simulink model "Model"  (R2023b)
settings: Solver=ode4  StartTime=0.0  StopTime=inf  FixedStep=1e-3  RelTol=1e-3
undefined symbols (not defined in the file): Actuatorparams, Aeroparams, Aircraftparams, Atmosphereparams, Earth, Inertiaconstants, Initialconds, Propparams, WGS84
libraries: simulink_extras x29, aerolibfltsims x2, aerolibtransform2 x1, vrlib x1
(part 1 of 3)
settings Model: Creator=bilal  LastModifiedBy=bilal
settings DebuggingCC: BusObjectLabelMismatch=error

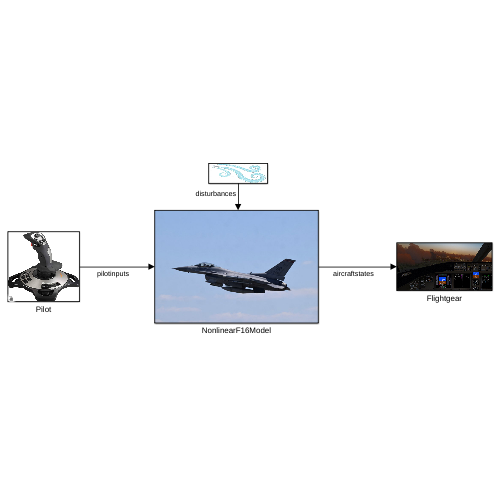
[thumbnail: Simulink's stored preview of the top-level diagram]
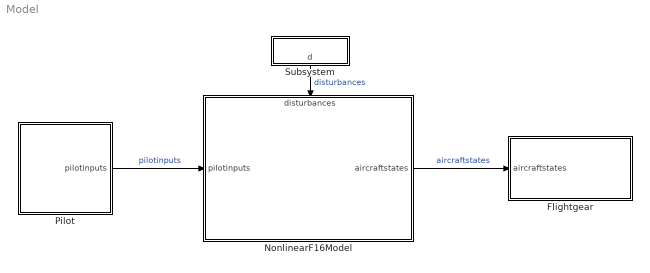
== system Model ==
  Flightgear : Subsystem
      mask Display: image('flightgear.jpg');
  NonlinearF16Model : Subsystem
      settings: PortSchema="{\"entries\":[{\"content\":{\"sides\":[{\"content\":{\"connectorIds\":[\"In1\"]},\"type\":\"ConnectorPlacement.EquallySpacedRectSide\",\"uuid\":\"b6fae004-6bc9-43de-a584-fcbf29e22be7\"},{\"content\":{\"connectorIds\":[\"Out1\"],\"side\":\"RIGHT\"},\"type\":\"ConnectorPlacement.EquallySpacedRectSide\",\"uuid\":\"50eeeff7-cc9e-45ad-978f-3a1c4ba7fd3d\"},{\"content\":{\"connectorIds\":[\"In2\"],\"side\":\"TOP\"},\"type\":\"ConnectorPlacement.EquallySpacedRectSide\",\"uuid\":\"669eaa38-3e90-4fd8-9c1d-c16541f97941\"}]},\"type\":\"ConnectorPlacement.EquallySpacedConnector\",\"uuid\":\"be7d5b6d-756e-471d-af56-7628ad948b10\"}],\"packageUris\":[\"http://schema.mathworks.com/mf0/Connector/R2020b\"],\"version\":\"1.0\"}"
      mask Display: image('f16.jpg');
  Pilot : Subsystem  Variant=on  VariantControlMode=label  LabelModeActiveChoice=pilotmode=manual
      mask Display: image('joystick.jpg');
  Subsystem : Subsystem
      mask Display: image('disturbance.png');
  wires:
  Pilot/1(pilotinputs) -> NonlinearF16Model/1(pilotinputs)  "pilotinputs"
  Subsystem/1(d) -> NonlinearF16Model/2(disturbances)  "disturbances"
  NonlinearF16Model/1(aircraftstates) -> Flightgear/1(aircraftstates)  "aircraftstates"

== system Model/Flightgear ==
  note: Instructions to setup FlightGear
      | Install FlightGear .
      | Open 'Generate Run Script' on the right.
      | On the Flightgear tab type your aircraft model name in 'FlightGear geometry model name'.
      | - Recommended model: 'c172p' as FlightGear
      | installes it by default.
      | - Additional aircrafts can be downloaded then.
      | On the File FlightGear base directory.
      | Click Generate Script.
      | Run generated script in Command Prompt (Windows) or in Terminal (Linux/macOS).
  aircraftstates : Inport
  Bus Selector : BusSelector  OutputSignals=rigidbodystates.positions.xe,rigidbodystates.positions.ye,rigidbodystates.positions.ze,rigidbodystates.eulerangles.phi,rigidbodystates.eulerangles.theta,rigidbodystates.eulerangles.psi
  Constant : Constant  Value=Initialconds.zeic
  Demux : Demux  Outputs=2
  Flat Earth to LLA : aerolibtransform2/Flat Earth to LLA  units=Metric (MKS)  ptype=Earth (WGS84)  F=1/298.257223563  R=6378137  refPosPort=off  LL0=[0 10]  psi=0
  FlightGear Preconfigured 6DoF Animation : aerolibfltsims/FlightGear Preconfigured 6DoF Animation  xFlightGearVersion=v2019.1  DestinationIpAddress=127.0.0.1  DestinationPort=5502  SampleTime=1e-3  packetVersion=24
  Flip : DSPFlip
  Generate Run Script : aerolibfltsims/Generate Run Script  Architecture=Default  dataFlow=Send  GeometryModelName=c172p  AirportId=KSFO  RunwayId=10L  InitialAltitude=7224  InitialHeading=113  OffsetDistance=4.72  OffsetAzimuth=0  InstallScenery=off  DisableShaders=off  OriginAddress=127.0.0.1  DestinationPort=5502  OriginPort=5505  LocalAddress=127.0.0.1  OutputFileName=runfg.bat  FlightGearBaseDirectory=C:\Program Files\FlightGear
  Mux : Mux  Inputs=3
  Mux1 : Mux  Inputs=6
  wires:
  aircraftstates/1 -> Bus Selector/1
  Bus Selector/2 -> Mux/2  "<ye>"
  Bus Selector/1 -> Mux/1  "<xe>"
  Bus Selector/3 -> Mux/3  "<ze>"
  Mux/1 -> Flat Earth to LLA/1
  Bus Selector/4 -> Mux1/4  "<phi>"
  Bus Selector/5 -> Mux1/5  "<theta>"
  Bus Selector/6 -> Mux1/6  "<psi>"
  Flat Earth to LLA/1 -> Flip/1
  Flip/1 -> Demux/1
  Demux/1 -> Mux1/1
  Demux/2 -> Mux1/2
  Flat Earth to LLA/2 -> Mux1/3
  Mux1/1 -> FlightGear Preconfigured 6DoF Animation/1
  Constant/1 -> Flat Earth to LLA/2

== system Model/NonlinearF16Model ==
  pilotinputs : Inport  OutDataTypeStr=Bus: pilotinputs
  disturbances : Inport  Port=2  OutDataTypeStr=Bus: disturbances
  Airframe : Subsystem
  Simframe : Subsystem
  aircraftstates : Outport  OutDataTypeStr=Bus: aircraftstates
  wires:
  pilotinputs/1 -> Airframe/1(pilotinputs)  "pilotinputs"
  Airframe/1(totalforces) -> Simframe/1(totalforces)
  Airframe/3(totalmoments) -> Simframe/3(totalmoments)
  Simframe/3(pressure) -> Airframe/4(pressure)  "pressure"
  Simframe/2(vtalphabeta) -> Airframe/3(vtalphabeta)  "vtalphabeta"
  Simframe/4(machheight) -> Airframe/5(machheight)  "machheight"
  disturbances/1 -> Simframe/2(disturbances)
  Simframe/1(rigidbodystates) -> Airframe/2(rigidbodystates)  "rigidbodystates"
  Airframe/2(aircraftstates) -> aircraftstates/1

== system Model/Pilot ==
  note: To change input mode click on variant subsystem and select in the menu above
  Joystickinput : Subsystem  VariantControl=pilotmode=joystick
  Manualinput : Subsystem  VariantControl=pilotmode=manual
  pilotinputs : Outport

== system Model/Subsystem ==
  Bus Creator : BusCreator  Inputs=3  OutDataTypeStr=Bus: disturbances
  Constant : Constant  Value=0
  Constant1 : Constant  Value=0
  Constant2 : Constant  Value=0
  d : Outport  OutDataTypeStr=Bus: disturbances
  wires:
  Constant1/1 -> Bus Creator/2  "windy"
  Constant/1 -> Bus Creator/1  "windx"
  Constant2/1 -> Bus Creator/3  "windz"
  Bus Creator/1 -> d/1

== system Model/NonlinearF16Model/Airframe ==
  pilotinputs : Inport  OutDataTypeStr=Bus: pilotinputs
  rigidbodystates : Inport  Port=2  OutDataTypeStr=Bus: rigidbodystates
  vtalphabeta : Inport  Port=3  OutDataTypeStr=Bus: vtalphabeta
  pressure : Inport  Port=4  OutDataTypeStr=Bus: pressure
  machheight : Inport  Port=5  OutDataTypeStr=Bus: machheight
  Actuator : Subsystem  mask{aileronslowerdeflectionlimit=Actuatorparams.aileronslowerdeflectionlimit, aileronsupperdeflectionlimit=Actuatorparams.aileronsupperdeflectionlimit, aileronslowerratelimit=Actuatorparams.aileronslowerratelimit, aileronsupperratelimit=Actuatorparams.aileronsupperratelimit, aileronstimeconstant=Actuatorparams.aileronstimeconstant, aileronsinitialvalue=Actuatorparams.aileronsinitialvalue, elevatorlowerdeflectionlimit=Actuatorparams.elevatorlowerdeflectionlimit, elevatorupperdeflectionlimit=Actuatorparams.elevatorupperdeflectionlimit, elevatorlowerratelimit=Actuatorparams.elevatorlowerratelimit, elevatorupperratelimit=Actuatorparams.elevatorupperratelimit, elevatortimeconstant=Actuatorparams.elevatortimeconstant, elevatorinitialvalue=Actuatorparams.elevatorinitialvalue, rudderlowerdeflectionlimit=Actuatorparams.rudderlowerdeflectionlimit, rudderupperdeflectionlimit=Actuatorparams.rudderupperdeflectionlimit, rudderlowerratelimit=Actuatorparams.rudderlowerratelimit, rudderupperratelimit=Actuatorparams.rudderupperratelimit, ruddertimeconstant=Actuatorparams.ruddertimeconstant, rudderinitialvalue=Actuatorparams.rudderinitialvalue, speedbrakelowerdeflectionlimit=Actuatorparams.speedbrakelowerdeflectionlimit, speedbrakeupperdeflectionlimit=Actuatorparams.speedbrakeupperdeflectionlimit}
      mask DialogControl DescTextVar Prompt: Actuator parameters for ailerons, elevator, rudder, and speed brake.
  Aerodynamic : Subsystem
  Bus Creator : BusCreator  Inputs=3  OutDataTypeStr=Bus: totalforces
  Bus Creator1 : BusCreator  Inputs=3  OutDataTypeStr=Bus: totalmoments
  Bus Creator2 : BusCreator  Inputs=2  OutDataTypeStr=Bus: aircraftstates
  Bus Selector : BusSelector  OutputSignals=actuatoraerooutputs,actuatorpropoutputs
  Bus Selector1 : BusSelector  OutputSignals=eulerangles,angularrates
  Mass : Subsystem
  Propulsion : Subsystem
  Sumforcesandmoments : Subsystem
  totalforces : Outport  OutDataTypeStr=Bus: totalforces
  aircraftstates : Outport  Port=2  OutDataTypeStr=Bus: aircraftstates
  totalmoments : Outport  Port=3  OutDataTypeStr=Bus: totalmoments
  wires:
  vtalphabeta/1 -> Aerodynamic/1(vtalphabeta)  "vtalphabeta"
  pressure/1 -> Aerodynamic/2(pressure)  "pressure"
  pilotinputs/1 -> Actuator/1(pilotinputs)
  Bus Selector/1 -> Aerodynamic/4(actuatoraerooutputs)  "<actuatoraerooutputs>"
  Bus Selector/2 -> Propulsion/1(actuatorpropoutputs)  "<actuatorpropoutputs>"
  Actuator/1(actuatoroutputs) -> Bus Selector/1
  machheight/1 -> Propulsion/3(machheight)  "machheight"
  Mass/1(massforces) -> Sumforcesandmoments/1(massforces)
  Aerodynamic/1(aeroforces) -> Sumforcesandmoments/2(aeroforces)
  Aerodynamic/2(aeromoments) -> Sumforcesandmoments/3(aeromoments)
  Propulsion/1(propforces) -> Sumforcesandmoments/4(propforces)
  Propulsion/2(propmoments) -> Sumforcesandmoments/5(propmoments)
  Sumforcesandmoments/2(Out2) -> Bus Creator/2  "Fy"
  Sumforcesandmoments/1(Out1) -> Bus Creator/1  "Fx"
  Sumforcesandmoments/3(Out3) -> Bus Creator/3  "Fz"
  Sumforcesandmoments/5(Out5) -> Bus Creator1/2  "My"
  Sumforcesandmoments/4(Out4) -> Bus Creator1/1  "Mx"
  Sumforcesandmoments/6(Out6) -> Bus Creator1/3  "Mz"
  Bus Creator/1 -> totalforces/1
  Bus Creator1/1 -> totalmoments/1
  rigidbodystates/1 -> Bus Creator2/1, Bus Selector1/1  "rigidbodystates"
  Bus Selector1/1 -> Mass/1(eulerangles)  "<eulerangles>"
  Bus Selector1/2 -> Aerodynamic/3(angularrates), Propulsion/2(angularrates)  "<angularrates>"
  Propulsion/3(enginestate) -> Bus Creator2/2  "enginestate"
  Bus Creator2/1 -> aircraftstates/1

== system Model/NonlinearF16Model/Simframe ==
  totalforces : Inport  OutDataTypeStr=Bus: totalforces
  disturbances : Inport  Port=2  OutDataTypeStr=Bus: disturbances
  totalmoments : Inport  Port=3  OutDataTypeStr=Bus: totalmoments
  Bus Creator : BusCreator  Inputs=4  OutDataTypeStr=Bus: rigidbodystates
  Environmentmodel : Subsystem
      settings: PortSchema="{\"entries\":[{\"content\":{\"sides\":[{\"content\":{\"connectorIds\":[\"In1\",\"In2\"]},\"type\":\"ConnectorPlacement.EquallySpacedRectSide\",\"uuid\":\"b6fae004-6bc9-43de-a584-fcbf29e22be7\"},{\"content\":{\"connectorIds\":[\"Out1\",\"Out2\",\"Out3\"],\"side\":\"RIGHT\"},\"type\":\"ConnectorPlacement.EquallySpacedRectSide\",\"uuid\":\"50eeeff7-cc9e-45ad-978f-3a1c4ba7fd3d\"},{\"content\":{\"connectorIds\":[\"In3\"],\"side\":\"TOP\"},\"type\":\"ConnectorPlacement.EquallySpacedRectSide\",\"uuid\":\"669eaa38-3e90-4fd8-9c1d-c16541f97941\"}]},\"type\":\"ConnectorPlacement.EquallySpacedConnector\",\"uuid\":\"be7d5b6d-756e-471d-af56-7628ad948b10\"}],\"packageUris\":[\"http://schema.mathworks.com/mf0/Connector/R2020b\"],\"version\":\"1.0\"}"
  Rigidbodydynamics : Subsystem
  rigidbodystates : Outport  OutDataTypeStr=Bus: rigidbodystates
  vtalphabeta : Outport  Port=2  OutDataTypeStr=Bus: vtalphabeta
  pressure : Outport  Port=3  OutDataTypeStr=Bus: pressure
  machheight : Outport  Port=4  OutDataTypeStr=Bus: machheight
  wires:
  totalforces/1 -> Rigidbodydynamics/1(totalforces)
  totalmoments/1 -> Rigidbodydynamics/2(totalmoments)
  Rigidbodydynamics/3(angularrates) -> Bus Creator/3  "angularrates"
  Rigidbodydynamics/2(eulerangles) -> Bus Creator/2  "eulerangles"
  Rigidbodydynamics/1(bodyvelocities) -> Environmentmodel/1(bodyvelocities), Bus Creator/1  "bodyvelocities"
  Rigidbodydynamics/4(positions) -> Environmentmodel/2(positions), Bus Creator/4  "positions"
  disturbances/1 -> Environmentmodel/3(disturbances)
  Environmentmodel/1(vtalphabeta) -> vtalphabeta/1
  Environmentmodel/2(pressure) -> pressure/1
  Environmentmodel/3(machheight) -> machheight/1
  Bus Creator/1 -> rigidbodystates/1

== system Model/Pilot/Joystickinput ==
  note: Thrust input can also be provided through Joystick with the appropriate device!
  Bus Creator : BusCreator  Inputs=5  OutDataTypeStr=Bus: pilotinputs
  Demux : Demux
  Joystick Input : vrlib/Joystick Input  joyid=1  adjustports=on  forcefeed=off
  Selector : Selector  InputPortWidth=8  IndexOptions=Index vector (dialog)  Indices=[1 2 4 7]  OutputSizes=1
  Terminator : Terminator
  Thrust : KnobBlock  LabelPosition=Hide  ScaleMax=1  TickInterval=0.1
  thrust : Constant  OutDataTypeStr=double
  pilotinputs : Outport  OutDataTypeStr=Bus: pilotinputs
  wires:
  Joystick Input/2 -> Terminator/1
  Joystick Input/1 -> Selector/1
  thrust/1 -> Bus Creator/5  "thrust"
  Demux/3 -> Bus Creator/3  "rudder"
  Selector/1 -> Demux/1
  Demux/1 -> Bus Creator/1  "ailerons"
  Demux/2 -> Bus Creator/2  "elevator"
  Demux/4 -> Bus Creator/4  "speedbrake"
  Bus Creator/1 -> pilotinputs/1  "pilotinputs"

== system Model/Pilot/Manualinput ==
  Ailerons : KnobBlock  LabelPosition=Hide  ScaleMin=-1  ScaleMax=1
  Bus Creator : BusCreator  Inputs=5  OutDataTypeStr=Bus: pilotinputs
  Elevator : KnobBlock  LabelPosition=Hide  ScaleMin=-1  ScaleMax=1
  Rudder : KnobBlock  LabelPosition=Hide  ScaleMin=-1  ScaleMax=1
  Thrust : KnobBlock  LabelPosition=Hide  ScaleMax=1  TickInterval=0.1
  ailerons : Constant  Value=0  OutDataTypeStr=double
  elevator : Constant  Value=0.0633840644587883  OutDataTypeStr=double
  rudder : Constant  Value=0  OutDataTypeStr=double
  speedbrake : Constant  Value=0  OutDataTypeStr=double
  thrust : Constant  Value=0.40277481430381  OutDataTypeStr=double
  pilotinputs : Outport  OutDataTypeStr=Bus: pilotinputs
  wires:
  thrust/1 -> Bus Creator/5  "thrust"
  rudder/1 -> Bus Creator/3  "rudder"
  Bus Creator/1 -> pilotinputs/1  "pilotinputs"
  ailerons/1 -> Bus Creator/1  "ailerons"
  elevator/1 -> Bus Creator/2  "elevator"
  speedbrake/1 -> Bus Creator/4  "speedbrake"

== system Model/NonlinearF16Model/Airframe/Actuator ==
  pilotinputs : Inport  OutDataTypeStr=Bus: pilotinputs
  Bus Creator : BusCreator  Inputs=4  OutDataTypeStr=Bus: actuatoraerooutputs
  Bus Creator1 : BusCreator  Inputs=1  OutDataTypeStr=Bus: actuatorpropoutputs
  Bus Creator2 : BusCreator  Inputs=2  OutDataTypeStr=Bus: actuatoroutputs
  Bus Selector : BusSelector  OutputSignals=ailerons,elevator,rudder,speedbrake,thrust
  Gain : Gain  Gain=-21.5
  Gain1 : Gain  Gain=-25
  Gain2 : Gain  Gain=-30
  Gain3 : Gain  Gain=60
  Gain4 : Gain
  Rate Limiter : RateLimiter  RisingSlewLimit=aileronsupperratelimit  FallingSlewLimit=aileronslowerratelimit
  Rate Limiter1 : RateLimiter  RisingSlewLimit=elevatorupperratelimit  FallingSlewLimit=elevatorlowerratelimit
  Rate Limiter2 : RateLimiter  RisingSlewLimit=rudderupperratelimit  FallingSlewLimit=rudderlowerratelimit
  Saturation : Saturate  UpperLimit=aileronsupperdeflectionlimit  LowerLimit=aileronslowerdeflectionlimit
  Saturation1 : Saturate  UpperLimit=elevatorupperdeflectionlimit  LowerLimit=elevatorlowerdeflectionlimit
  Saturation2 : Saturate  UpperLimit=rudderupperdeflectionlimit  LowerLimit=rudderlowerdeflectionlimit
  Saturation3 : Saturate  UpperLimit=speedbrakeupperdeflectionlimit  LowerLimit=speedbrakelowerdeflectionlimit
  Transfer Fcn (with initial states) : simulink_extras/Additional Linear/Transfer Fcn (with initial states)  N=[1]  D=[aileronstimeconstant 1]  X0=aileronsinitialvalue
  Transfer Fcn (with initial states)1 : simulink_extras/Additional Linear/Transfer Fcn (with initial states)  N=[1]  D=[elevatortimeconstant 1]  X0=elevatorinitialvalue
  Transfer Fcn (with initial states)2 : simulink_extras/Additional Linear/Transfer Fcn (with initial states)  N=[1]  D=[ruddertimeconstant 1]  X0=rudderinitialvalue
  actuatoroutputs : Outport  OutDataTypeStr=Bus: actuatoroutputs
  wires:
  pilotinputs/1 -> Bus Selector/1
  Bus Selector/1 -> Gain/1  "<ailerons>"
  Bus Selector/2 -> Gain1/1  "<elevator>"
  Bus Selector/3 -> Gain2/1  "<rudder>"
  Bus Selector/4 -> Gain3/1  "<speedbrake>"
  Bus Selector/5 -> Gain4/1  "<thrust>"
  Gain/1 -> Saturation/1
  Gain1/1 -> Saturation1/1
  Gain2/1 -> Saturation2/1
  Gain3/1 -> Saturation3/1
  Saturation/1 -> Rate Limiter/1
  Saturation1/1 -> Rate Limiter1/1
  Saturation2/1 -> Rate Limiter2/1
  Saturation3/1 -> Bus Creator/4  "speedbrake"
  Gain4/1 -> Bus Creator1/1  "thrust"
  Rate Limiter/1 -> Transfer Fcn (with initial states)/1
  Rate Limiter1/1 -> Transfer Fcn (with initial states)1/1
  Rate Limiter2/1 -> Transfer Fcn (with initial states)2/1
  Transfer Fcn (with initial states)2/1 -> Bus Creator/3  "rudder"
  Transfer Fcn (with initial states)1/1 -> Bus Creator/2  "elevator"
  Transfer Fcn (with initial states)/1 -> Bus Creator/1  "ailerons"
  Bus Creator/1 -> Bus Creator2/1  "actuatoraerooutputs"
  Bus Creator1/1 -> Bus Creator2/2  "actuatorpropoutputs"
  Bus Creator2/1 -> actuatoroutputs/1

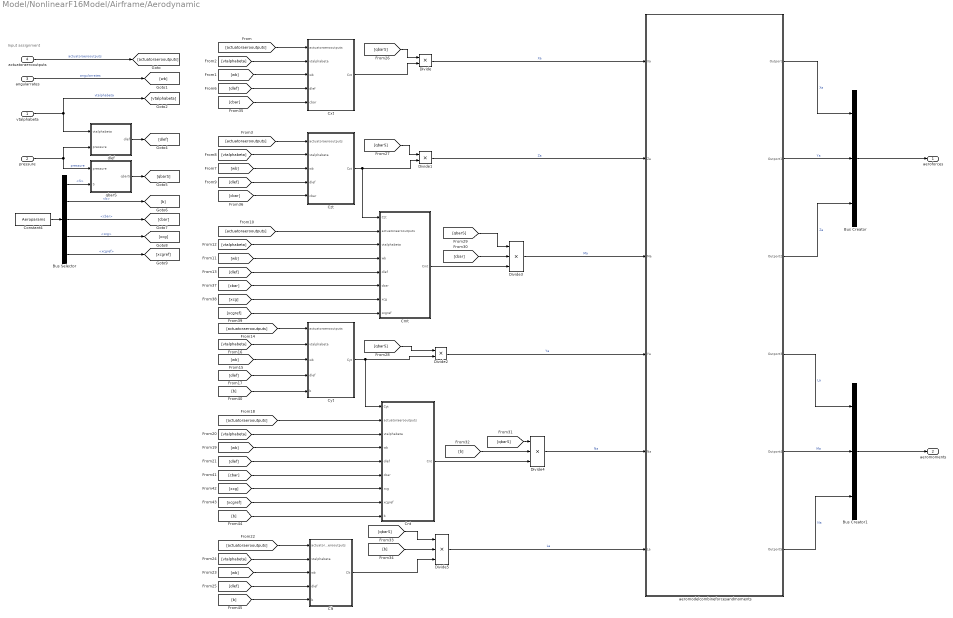
== system Model/NonlinearF16Model/Airframe/Aerodynamic ==
  note: Input assignment
  vtalphabeta : Inport  OutDataTypeStr=Bus: vtalphabeta
  pressure : Inport  Port=2  OutDataTypeStr=Bus: pressure
  angularrates : Inport  Port=3  OutDataTypeStr=Bus: angularrates
  actuatoraerooutputs : Inport  Port=4  OutDataTypeStr=Bus: actuatoraerooutputs
  Bus Creator : BusCreator  Inputs=3
  Bus Creator1 : BusCreator  Inputs=3
  Bus Selector : BusSelector  OutputSignals=S,b,cbar,xcg,xcgref
  Clt : Subsystem
  Cmt : Subsystem
  Cnt : Subsystem
  Constant4 : Constant  Value=Aeroparams  OutDataTypeStr=Bus: aeroparams
  Cxt : Subsystem
  Cyt : Subsystem
  Czt : Subsystem
  Divide : Product  Inputs=**
  Divide1 : Product  Inputs=**
  Divide2 : Product  Inputs=**
  Divide3 : Product  Inputs=***
  Divide4 : Product  Inputs=***
  Divide5 : Product  Inputs=***
  aeromodelcombineforcesandmoments : Subsystem
  dlef : Subsystem  mask{leflowerdeflectionlimit=Actuatorparams.leflowerdeflectionlimit, lefupperdeflectionlimit=Actuatorparams.lefupperdeflectionlimit, leflowerratelimit=Actuatorparams.leflowerratelimit, lefupperratelimit=Actuatorparams.lefupperratelimit, leftimeconstant=Actuatorparams.leftimeconstant, lefinitialvalue=Actuatorparams.lefinitialvalue}
      mask DialogControl DescTextVar Prompt: Leading edge flap paramaters
  qbarS : Subsystem
  aeroforces : Outport  OutDataTypeStr=Bus: aeroforces
  aeromoments : Outport  Port=2  OutDataTypeStr=Bus: aeromoments
  wires:
  actuatoraerooutputs/1 -> [actuatoraerooutputs]  "actuatoraerooutputs"
  angularrates/1 -> [wb]  "angularrates"
  vtalphabeta/1 -> dlef/1(vtalphabeta), [vtalphabeta]  "vtalphabeta"
  pressure/1 -> dlef/2(pressure), qbarS/1(pressure)  "pressure"
  dlef/1(dlef) -> [dlef]
  [vtalphabeta] -> Cxt/2(vtalphabeta)
  [actuatoraerooutputs] -> Cxt/1(actuatoraerooutputs)
  [wb] -> Cxt/3(wb)
  [dlef] -> Cxt/4(dlef)
  [dlef] -> Czt/4(dlef)
  [wb] -> Czt/3(wb)
  [actuatoraerooutputs] -> Czt/1(actuatoraerooutputs)
  [vtalphabeta] -> Czt/2(vtalphabeta)
  [vtalphabeta] -> Cmt/3(vtalphabeta)
  [actuatoraerooutputs] -> Cmt/2(actuatoraerooutputs)
  [wb] -> Cmt/4(wb)
  [dlef] -> Cmt/5(dlef)
  [dlef] -> Cyt/4(dlef)
  [wb] -> Cyt/3(wb)
  [actuatoraerooutputs] -> Cyt/1(actuatoraerooutputs)
  [vtalphabeta] -> Cyt/2(vtalphabeta)
  [vtalphabeta] -> Cnt/3(vtalphabeta)
  [actuatoraerooutputs] -> Cnt/2(actuatoraerooutputs)
  [wb] -> Cnt/4(wb)
  [dlef] -> Cnt/5(dlef)
  Cyt/1(Cyt) -> Divide2/2, Cnt/1(Cyt)
  [dlef] -> Clt/4(dlef)
  [wb] -> Clt/3(wb)
  [actuatoraerooutputs] -> Clt/1(actuatoraerooutputs)
  [vtalphabeta] -> Clt/2(vtalphabeta)
  qbarS/1(qbarS) -> [qbarS]
  [qbarS] -> Divide/1
  Cxt/1(Cxt) -> Divide/2
  Czt/1(Czt) -> Divide1/2, Cmt/1(Czt)
  [qbarS] -> Divide1/1
  [qbarS] -> Divide2/1
  [qbarS] -> Divide3/1
  [cbar] -> Divide3/2
  Cmt/1(Cmt) -> Divide3/3
  Cnt/1(Cnt) -> Divide4/3
  [b] -> Divide4/2
  [qbarS] -> Divide4/1
  [qbarS] -> Divide5/1
  [b] -> Divide5/2
  Clt/1(Clt) -> Divide5/3
  Divide/1 -> aeromodelcombineforcesandmoments/1(Xa)  "Xa"
  Divide1/1 -> aeromodelcombineforcesandmoments/2(Za)  "Za"
  Divide3/1 -> aeromodelcombineforcesandmoments/3(Ma)  "Ma"
  Divide2/1 -> aeromodelcombineforcesandmoments/4(Ya)  "Ya"
  Divide4/1 -> aeromodelcombineforcesandmoments/5(Na)  "Na"
  Divide5/1 -> aeromodelcombineforcesandmoments/6(La)  "La"
  Constant4/1 -> Bus Selector/1
  Bus Selector/1 -> qbarS/2(S)  "<S>"
  Bus Selector/2 -> [b]  "<b>"
  Bus Selector/3 -> [cbar]  "<cbar>"
  Bus Selector/4 -> [xcg]  "<xcg>"
  Bus Selector/5 -> [xcgref]  "<xcgref>"
  [cbar] -> Cxt/5(cbar)
  [cbar] -> Czt/5(cbar)
  [cbar] -> Cmt/6(cbar)
  [xcg] -> Cmt/7(xcg)
  [xcgref] -> Cmt/8(xcgref)
  [b] -> Cyt/5(b)
  [b] -> Cnt/9(b)
  [xcgref] -> Cnt/8(xcgref)
  [xcg] -> Cnt/7(xcg)
  [cbar] -> Cnt/6(cbar)
  [b] -> Clt/5(b)
  aeromodelcombineforcesandmoments/2(Outport1) -> Bus Creator/2  "Ya"
  aeromodelcombineforcesandmoments/1(Outport) -> Bus Creator/1  "Xa"
  aeromodelcombineforcesandmoments/3(Outport2) -> Bus Creator/3  "Za"
  aeromodelcombineforcesandmoments/5(Outport4) -> Bus Creator1/2  "Ma"
  aeromodelcombineforcesandmoments/4(Outport3) -> Bus Creator1/1  "La"
  aeromodelcombineforcesandmoments/6(Outport5) -> Bus Creator1/3  "Na"
  Bus Creator1/1 -> aeromoments/1
  Bus Creator/1 -> aeroforces/1

== system Model/NonlinearF16Model/Airframe/Mass ==
  eulerangles : Inport  OutDataTypeStr=Bus: eulerangles
  Bus Creator : BusCreator  Inputs=3
  Bus Selector : BusSelector  OutputSignals=m
  Bus Selector1 : BusSelector  OutputSignals=phi,theta,psi
  Constant : Constant  Value=Aircraftparams  OutDataTypeStr=Bus: aircraftparams
  Divide : Product  Inputs=**
  Selector : Selector  InputPortWidth=3  IndexOptions=Index vector (dialog)  Indices=1  OutputSizes=1
  Selector1 : Selector  InputPortWidth=3  IndexOptions=Index vector (dialog)  Indices=2  OutputSizes=1
  Selector2 : Selector  InputPortWidth=3  IndexOptions=Index vector (dialog)  Indices=3  OutputSizes=1
  massmodelgb : Subsystem
  massforces : Outport  OutDataTypeStr=Bus: massforces
  wires:
  Constant/1 -> Bus Selector/1
  eulerangles/1 -> Bus Selector1/1
  Bus Selector1/1 -> massmodelgb/1(<phi>)  "<phi>"
  Bus Selector1/2 -> massmodelgb/2(<theta>)  "<theta>"
  Bus Selector1/3 -> massmodelgb/3(<psi>)  "<psi>"
  massmodelgb/1(gb) -> Divide/1
  Selector/1 -> Bus Creator/1  "Fgx"
  Divide/1 -> Selector/1, Selector1/1, Selector2/1
  Bus Creator/1 -> massforces/1
  Bus Selector/1 -> Divide/2  "<m>"
  Selector1/1 -> Bus Creator/2  "Fgy"
  Selector2/1 -> Bus Creator/3  "Fgz"

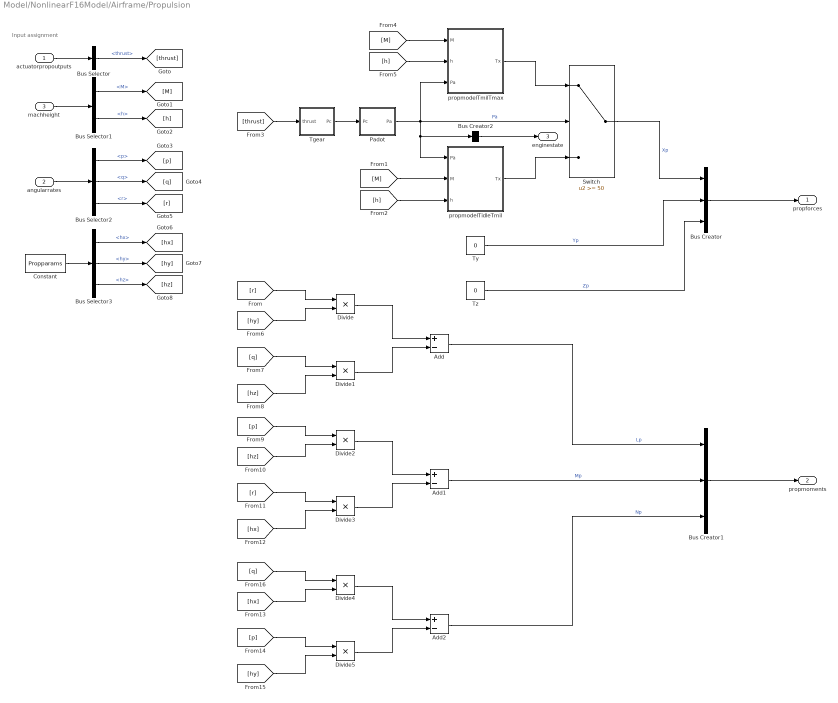
== system Model/NonlinearF16Model/Airframe/Propulsion ==
  note: Input assignment
  actuatorpropoutputs : Inport  OutDataTypeStr=Bus: actuatorpropoutputs
  angularrates : Inport  Port=2
  machheight : Inport  Port=3
  Add : Sum  Inputs=+-
  Add1 : Sum  Inputs=+-
  Add2 : Sum  Inputs=+-
  Bus Creator : BusCreator  Inputs=3  OutDataTypeStr=Bus: propforces
  Bus Creator1 : BusCreator  Inputs=3  OutDataTypeStr=Bus: propmoments
  Bus Creator2 : BusCreator  Inputs=1  OutDataTypeStr=Bus: enginestate
  Bus Selector : BusSelector  OutputSignals=thrust
  Bus Selector1 : BusSelector  OutputSignals=M,h
  Bus Selector2 : BusSelector  OutputSignals=p,q,r
  Bus Selector3 : BusSelector  OutputSignals=hx,hy,hz
  Constant : Constant  Value=Propparams  OutDataTypeStr=Bus: propparams
  Divide{,1..5} (6 alike) : Product  Inputs=**
  Padot : Subsystem
  Switch : Switch  Threshold=50  SaturateOnIntegerOverflow=off  InputSameDT=off
  Tgear : Subsystem
  Ty : Constant  Value=0
  Tz : Constant  Value=0
  propmodelTidleTmil : Subsystem
  propmodelTmilTmax : Subsystem
  propforces : Outport  OutDataTypeStr=Bus: propforces
  propmoments : Outport  Port=2  OutDataTypeStr=Bus: propmoments
  enginestate : Outport  Port=3  OutDataTypeStr=Bus: enginestate
  wires:
  actuatorpropoutputs/1 -> Bus Selector/1
  Tgear/1(Pc) -> Padot/1(Pc)
  Padot/1(Pa) -> Bus Creator2/1, propmodelTidleTmil/1(Pa), Switch/2, propmodelTmilTmax/3(Pa)  "Pa"
  machheight/1 -> Bus Selector1/1
  Bus Selector/1 -> [thrust]  "<thrust>"
  Bus Selector1/1 -> [M]  "<M>"
  Bus Selector1/2 -> [h]  "<h>"
  [M] -> propmodelTidleTmil/2(M)
  [h] -> propmodelTidleTmil/3(h)
  [thrust] -> Tgear/1(thrust)
  [h] -> propmodelTmilTmax/2(h)
  [M] -> propmodelTmilTmax/1(M)
  propmodelTmilTmax/1(Tx) -> Switch/1
  propmodelTidleTmil/1(Tx) -> Switch/3
  Switch/1 -> Bus Creator/1  "Xp"
  Ty/1 -> Bus Creator/2  "Yp"
  Tz/1 -> Bus Creator/3  "Zp"
  Bus Creator/1 -> propforces/1
  angularrates/1 -> Bus Selector2/1
  Bus Selector2/1 -> [p]  "<p>"
  Bus Selector2/2 -> [q]  "<q>"
  Bus Selector2/3 -> [r]  "<r>"
  Constant/1 -> Bus Selector3/1
  Bus Selector3/1 -> [hx]  "<hx>"
  Bus Selector3/2 -> [hy]  "<hy>"
  Bus Selector3/3 -> [hz]  "<hz>"
  [r] -> Divide/1
  [hy] -> Divide/2
  [q] -> Divide1/1
  [hz] -> Divide1/2
  Divide/1 -> Add/1
  Divide1/1 -> Add/2
  Divide3/1 -> Add1/2
  Divide2/1 -> Add1/1
  [hx] -> Divide3/2
  [r] -> Divide3/1
  [hz] -> Divide2/2
  [p] -> Divide2/1
  [q] -> Divide4/1
  [hx] -> Divide4/2
  [p] -> Divide5/1
  [hy] -> Divide5/2
  Divide4/1 -> Add2/1
  Divide5/1 -> Add2/2
  Add1/1 -> Bus Creator1/2  "Mp"
  Add/1 -> Bus Creator1/1  "Lp"
  Add2/1 -> Bus Creator1/3  "Np"
  Bus Creator1/1 -> propmoments/1
  Bus Creator2/1 -> enginestate/1

== system Model/NonlinearF16Model/Airframe/Sumforcesandmoments ==
  massforces : Inport
  aeroforces : Inport  Port=2
  aeromoments : Inport  Port=3
  propforces : Inport  Port=4
  propmoments : Inport  Port=5
  Add : Sum  Inputs=+++
  Add1 : Sum
  Demux : Demux  Outputs=3
  Demux1 : Demux  Outputs=3
  Out1 : Outport
  Out2 : Outport  Port=2
  Out3 : Outport  Port=3
  Out4 : Outport  Port=4
  Out5 : Outport  Port=5
  Out6 : Outport  Port=6
  wires:
  massforces/1 -> Add/1
  aeroforces/1 -> Add/2
  propforces/1 -> Add/3
  propmoments/1 -> Add1/2
  aeromoments/1 -> Add1/1
  Add/1 -> Demux/1
  Demux/1 -> Out1/1  "Fx"
  Demux/2 -> Out2/1  "Fy"
  Demux/3 -> Out3/1  "Fz"
  Add1/1 -> Demux1/1
  Demux1/1 -> Out4/1  "Mx"
  Demux1/2 -> Out5/1  "My"
  Demux1/3 -> Out6/1  "Mz"

== system Model/NonlinearF16Model/Simframe/Environmentmodel ==
  note: Input assignment
  bodyvelocities : Inport
  positions : Inport  Port=2
  disturbances : Inport  Port=3
  Bus Creator : BusCreator  Inputs=2  OutDataTypeStr=Bus: pressure
  Bus Creator2 : BusCreator  Inputs=3  OutDataTypeStr=Bus: vtalphabeta
  Bus Creator3 : BusCreator  Inputs=2  OutDataTypeStr=Bus: machheight
  Bus Selector : BusSelector  OutputSignals=L,T0,gamma,R,g0,rho0
  Bus Selector1 : BusSelector  OutputSignals=ze
  Constant : Constant  Value=Atmosphereparams  OutDataTypeStr=Bus: atmosphereparams
  Gain : Gain  Gain=-1
  Vtalphabeta : Subsystem
  envmodelTM : Subsystem
  envmodelqbarPs : Subsystem
  envmodelrho : Subsystem
  vtalphabeta : Outport  OutDataTypeStr=Bus: vtalphabeta
  pressure : Outport  Port=2  OutDataTypeStr=Bus: pressure
  machheight : Outport  Port=3  OutDataTypeStr=Bus: machheight
  wires:
  [R] -> envmodelqbarPs/2(R)
  envmodelrho/1(rho) -> envmodelqbarPs/1(rho)
  [rho0] -> envmodelrho/7(rho0)
  [h] -> envmodelrho/6(h)  "h"
  [R] -> envmodelrho/5(R)
  [L] -> envmodelrho/4(L)
  [g0] -> envmodelrho/3(g0)
  [T0] -> envmodelrho/2(T0)
  [T] -> envmodelrho/1(T)
  Bus Creator3/1 -> machheight/1
  [h] -> Bus Creator3/2  "h"
  envmodelTM/2(M) -> Bus Creator3/1
  [R] -> envmodelTM/5(R)
  [gamma] -> envmodelTM/4(gamma)
  envmodelTM/1(T) -> [T]
  [h] -> envmodelTM/3(h)
  [L] -> envmodelTM/2(L)
  [T0] -> envmodelTM/1(T0)
  Vtalphabeta/3(beta) -> Bus Creator2/3  "beta"
  Vtalphabeta/1(Vt) -> envmodelTM/6(Vt), envmodelqbarPs/4(Vt), Bus Creator2/1  "Vt"
  Vtalphabeta/2(alpha) -> Bus Creator2/2  "alpha"
  Bus Creator2/1 -> vtalphabeta/1
  bodyvelocities/1 -> Vtalphabeta/2(bodyvelocities)
  disturbances/1 -> Vtalphabeta/1(disturbances)
  Gain/1 -> [h]
  Bus Selector1/1 -> Gain/1  "<ze>"
  positions/1 -> Bus Selector1/1
  Bus Selector/6 -> [rho0]  "<rho0>"
  Bus Selector/5 -> [g0]  "<g0>"
  Bus Selector/4 -> [R]  "<R>"
  Bus Selector/3 -> [gamma]  "<gamma>"
  Bus Selector/2 -> [T0]  "<T0>"
  Bus Selector/1 -> [L]  "<L>"
  Constant/1 -> Bus Selector/1
  Bus Creator/1 -> pressure/1
  envmodelqbarPs/1(qbar) -> Bus Creator/1
  envmodelqbarPs/2(Ps) -> Bus Creator/2
  [T] -> envmodelqbarPs/3(T)

== system Model/NonlinearF16Model/Simframe/Rigidbodydynamics ==
  totalforces : Inport
  totalmoments : Inport  Port=2
  Forceequations : Subsystem
  Kinematicequations : Subsystem
  Momentequations : Subsystem
  Navigationequations : Subsystem
  bodyvelocities : Outport  OutDataTypeStr=Bus: bodyvelocities
  eulerangles : Outport  Port=2  OutDataTypeStr=Bus: eulerangles
  angularrates : Outport  Port=3  OutDataTypeStr=Bus: angularrates
  positions : Outport  Port=4  OutDataTypeStr=Bus: positions
  wires:
  totalforces/1 -> Forceequations/1(totalforces)
  totalmoments/1 -> Momentequations/1(totalmoments)
  Momentequations/1(angularrates) -> Kinematicequations/1(angularrates), angularrates/1, Forceequations/2(angularrates)
  Forceequations/1(bodyvelocities) -> bodyvelocities/1, Navigationequations/1(bodyvelocities)
  Kinematicequations/1(eulerangles) -> eulerangles/1, Navigationequations/2(eulerangles)
  Navigationequations/1(positions) -> positions/1

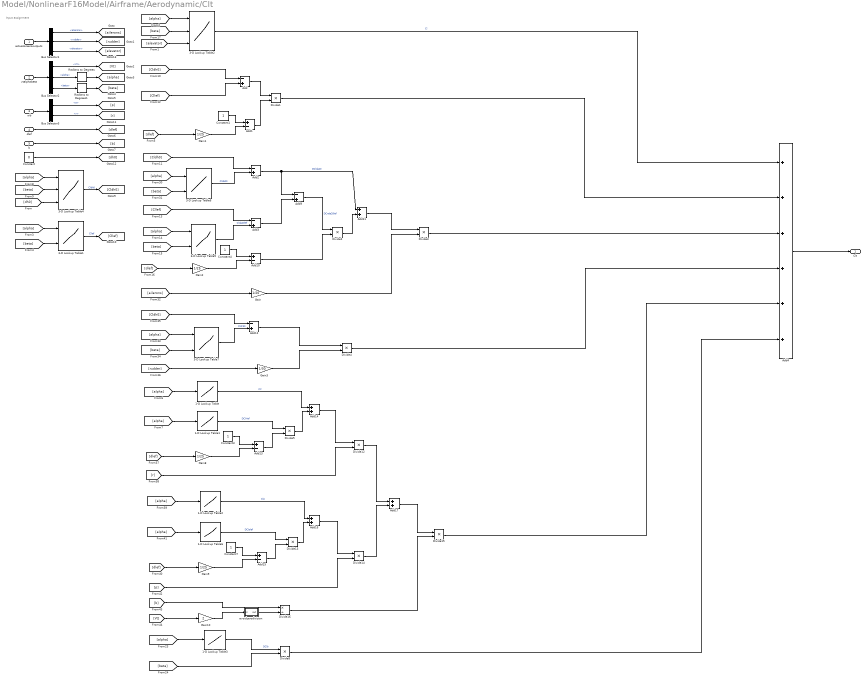
== system Model/NonlinearF16Model/Airframe/Aerodynamic/Clt ==
  note: Input assignment
  actuatoraerooutputs : Inport
  vtalphabeta : Inport  Port=2
  wb : Inport  Port=3
  dlef : Inport  Port=4
  b : Inport  Port=5
  1-D Lookup Table : Lookup_n-D  NumberOfTableDimensions=1  BreakpointsForDimension1=Aeroparams.alpha  Table=Aeroparams.Clr  InternalRulePriority=Speed  RndMeth=Simplest
  1-D Lookup Table1 : Lookup_n-D  NumberOfTableDimensions=1  BreakpointsForDimension1=Aeroparams.alpha(1:14)  Table=Aeroparams.DClrlef  InternalRulePriority=Speed  RndMeth=Simplest
  1-D Lookup Table2 : Lookup_n-D  NumberOfTableDimensions=1  BreakpointsForDimension1=Aeroparams.alpha  Table=Aeroparams.Clp  InternalRulePriority=Speed  RndMeth=Simplest
  1-D Lookup Table3 : Lookup_n-D  NumberOfTableDimensions=1  BreakpointsForDimension1=Aeroparams.alpha  Table=Aeroparams.DClb  InternalRulePriority=Speed  RndMeth=Simplest
  1-D Lookup Table6 : Lookup_n-D  NumberOfTableDimensions=1  BreakpointsForDimension1=Aeroparams.alpha(1:14)  Table=Aeroparams.DClplef  InternalRulePriority=Speed  RndMeth=Simplest
  3-D Lookup Table1 : Lookup_n-D  BreakpointsForDimension1=Aeroparams.alpha(1:14)  BreakpointsForDimension2=Aeroparams.beta  BreakpointsForDimension3=Aeroparams.dh  Table=Aeroparams.Cllef  InternalRulePriority=Speed  RndMeth=Simplest
      settings: InputPortMap=u0,u1
  3-D Lookup Table2 : Lookup_n-D  NumberOfTableDimensions=3  BreakpointsForDimension1=Aeroparams.alpha  BreakpointsForDimension2=Aeroparams.beta  BreakpointsForDimension3=Aeroparams.dh([1 3 5])  Table=Aeroparams.Cl  InternalRulePriority=Speed  RndMeth=Simplest
      settings: InputPortMap=u0,u1,u2
  3-D Lookup Table4 : Lookup_n-D  NumberOfTableDimensions=3  BreakpointsForDimension1=Aeroparams.alpha  BreakpointsForDimension2=Aeroparams.beta  BreakpointsForDimension3=Aeroparams.dh([1 3 5])  Table=Aeroparams.Cl  InternalRulePriority=Speed  RndMeth=Simplest
      settings: InputPortMap=u0,u1,u2
  3-D Lookup Table5 : Lookup_n-D  BreakpointsForDimension1=Aeroparams.alpha(1:14)  BreakpointsForDimension2=Aeroparams.beta  BreakpointsForDimension3=Aeroparams.dh  Table=Aeroparams.Clda20lef  InternalRulePriority=Speed  RndMeth=Simplest
      settings: InputPortMap=u0,u1
  3-D Lookup Table6 : Lookup_n-D  BreakpointsForDimension1=Aeroparams.alpha  BreakpointsForDimension2=Aeroparams.beta  BreakpointsForDimension3=Aeroparams.dh  Table=Aeroparams.Clda20  InternalRulePriority=Speed  RndMeth=Simplest
      settings: InputPortMap=u0,u1
  3-D Lookup Table7 : Lookup_n-D  BreakpointsForDimension1=Aeroparams.alpha  BreakpointsForDimension2=Aeroparams.beta  BreakpointsForDimension3=Aeroparams.dh  Table=Aeroparams.Cldr30  InternalRulePriority=Speed  RndMeth=Simplest
      settings: InputPortMap=u0,u1
  Add{,2..3,9,12} (5 alike) : Sum  Inputs=-+
  Add{1,10,13,15} (4 alike) : Sum  Inputs=+-
  Add{11,14,16..17} (4 alike) : Sum
  Add4 : Sum  Inputs=++++++
  Bus Selector1 : BusSelector  OutputSignals=ailerons,rudder,elevator
  Bus Selector2 : BusSelector  OutputSignals=Vt,alpha,beta
  Bus Selector3 : BusSelector  OutputSignals=p,r
  Constant : Constant  Value=0
  Constant{1,3..4,7} (4 alike) : Constant
  Divide{1..5,8,12..15} (10 alike) : Product  Inputs=**
  Divide16 : Product  Inputs=*/
  Gain : Gain  Gain=1/20
  Gain{1..2,8..9} (4 alike) : Gain  Gain=1/25
  Gain10 : Gain  Gain=2
  Gain3 : Gain  Gain=1/30
  Radians to Degrees : simulink_extras/Transformations/Radians to Degrees
  Radians to Degrees1 : simulink_extras/Transformations/Radians to Degrees
  avoidzerodivision : Subsystem
  Clt : Outport
  wires:
  [beta] -> Divide8/2
  1-D Lookup Table3/1 -> Divide8/1  "DClb"
  [alpha] -> 1-D Lookup Table3/1
  Bus Selector1/3 -> [elevator]  "<elevator>"
  [beta] -> 3-D Lookup Table2/2
  [alpha] -> 3-D Lookup Table2/1
  [elevator] -> 3-D Lookup Table2/3
  [dh0] -> 3-D Lookup Table4/3
  Constant/1 -> [dh0]
  Add4/1 -> Clt/1
  dlef/1 -> [dlef]
  Bus Selector3/1 -> [p]  "<p>"
  Bus Selector2/3 -> Radians to Degrees1/1  "<beta>"
  Bus Selector2/2 -> Radians to Degrees/1  "<alpha>"
  Bus Selector2/1 -> [Vt]  "<Vt>"
  Bus Selector1/2 -> [rudder]  "<rudder>"
  Bus Selector1/1 -> [ailerons]  "<ailerons>"
  wb/1 -> Bus Selector3/1
  vtalphabeta/1 -> Bus Selector2/1
  actuatoraerooutputs/1 -> Bus Selector1/1
  [Cllef] -> Add/2
  Gain1/1 -> Add1/2
  Constant1/1 -> Add1/1
  [dlef] -> Gain1/1
  Add/1 -> Divide1/1
  Add1/1 -> Divide1/2
  [alpha] -> 3-D Lookup Table4/1
  [beta] -> 3-D Lookup Table4/2
  3-D Lookup Table4/1 -> [Cldh0]  "Cldh0"
  [Cldh0] -> Add/1
  [Cldh0] -> Add2/1
  [beta] -> 3-D Lookup Table1/2
  [alpha] -> 3-D Lookup Table1/1
  3-D Lookup Table1/1 -> [Cllef]  "Cllef"
  [Cllef] -> Add3/1
  3-D Lookup Table5/1 -> Add3/2  "Clda20lef"
  [alpha] -> 3-D Lookup Table5/1
  [beta] -> 3-D Lookup Table5/2
  Add2/1 -> Add9/1, Add11/1  "DClda20"
  Add3/1 -> Add9/2
  3-D Lookup Table6/1 -> Add2/2  "Clda20"
  [beta] -> 3-D Lookup Table6/2
  [alpha] -> 3-D Lookup Table6/1
  Add9/1 -> Divide2/1  "DCnda20lef"
  Add10/1 -> Divide2/2
  [dlef] -> Gain2/1
  Constant4/1 -> Add10/1
  Gain2/1 -> Add10/2
  Divide2/1 -> Add11/2
  Add11/1 -> Divide3/1
  [ailerons] -> Gain/1
  Gain/1 -> Divide3/2
  [beta] -> 3-D Lookup Table7/2
  [alpha] -> 3-D Lookup Table7/1
  3-D Lookup Table7/1 -> Add12/2  "Cldr30"
  [Cldh0] -> Add12/1
  [rudder] -> Gain3/1
  Add12/1 -> Divide4/1
  Gain3/1 -> Divide4/2
  Bus Selector3/2 -> [r]  "<r>"
  [alpha] -> 1-D Lookup Table/1
  [alpha] -> 1-D Lookup Table1/1
  Gain8/1 -> Add13/2
  Constant3/1 -> Add13/1
  [dlef] -> Gain8/1
  Add13/1 -> Divide5/2
  1-D Lookup Table1/1 -> Divide5/1  "DClrlef"
  1-D Lookup Table/1 -> Add14/1  "Clr"
  Divide5/1 -> Add14/2
  Add14/1 -> Divide12/1
  [r] -> Divide12/2
  1-D Lookup Table2/1 -> Add16/1  "Clp"
  [alpha] -> 1-D Lookup Table2/1
  Divide13/1 -> Add16/2
  1-D Lookup Table6/1 -> Divide13/1  "DClplef"
  Add15/1 -> Divide13/2
  [dlef] -> Gain9/1
  Constant7/1 -> Add15/1
  Gain9/1 -> Add15/2
  [alpha] -> 1-D Lookup Table6/1
  Add16/1 -> Divide14/1
  [p] -> Divide14/2
  Divide12/1 -> Add17/1
  Divide14/1 -> Add17/2
  Add17/1 -> Divide15/1
  [b] -> Divide16/1
  [Vt] -> Gain10/1
  Gain10/1 -> avoidzerodivision/1(in)
  Divide16/1 -> Divide15/2
  3-D Lookup Table2/1 -> Add4/1  "Cl"
  Divide1/1 -> Add4/2
  Divide3/1 -> Add4/3
  Divide4/1 -> Add4/4
  Divide15/1 -> Add4/5
  Divide8/1 -> Add4/6
  b/1 -> [b]
  avoidzerodivision/1(out) -> Divide16/2
  Radians to Degrees/1 -> [alpha]
  Radians to Degrees1/1 -> [beta]

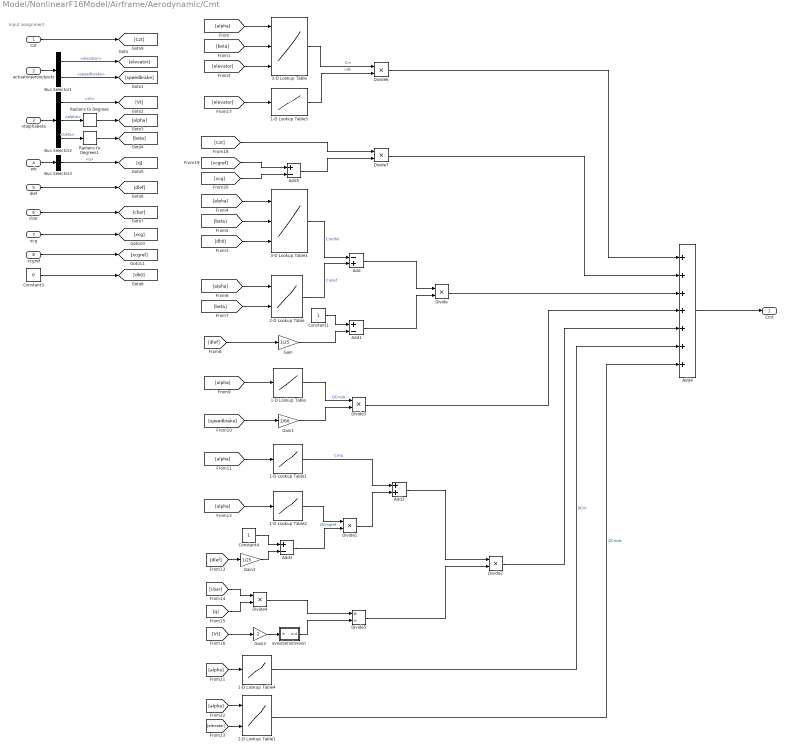
== system Model/NonlinearF16Model/Airframe/Aerodynamic/Cmt ==
  note: Input assignment
  Czt : Inport
  actuatoraerooutputs : Inport  Port=2
  vtalphabeta : Inport  Port=3
  wb : Inport  Port=4
  dlef : Inport  Port=5
  cbar : Inport  Port=6
  xcg : Inport  Port=7
  xcgref : Inport  Port=8
  1-D Lookup Table : Lookup_n-D  NumberOfTableDimensions=1  BreakpointsForDimension1=Aeroparams.alpha  Table=Aeroparams.DCmsb  InternalRulePriority=Speed  RndMeth=Simplest
  1-D Lookup Table1 : Lookup_n-D  NumberOfTableDimensions=1  BreakpointsForDimension1=Aeroparams.alpha  Table=Aeroparams.Cmq  InternalRulePriority=Speed  RndMeth=Simplest
  1-D Lookup Table2 : Lookup_n-D  NumberOfTableDimensions=1  BreakpointsForDimension1=Aeroparams.alpha(1:14)  Table=Aeroparams.DCmqlef  InternalRulePriority=Speed  RndMeth=Simplest
  1-D Lookup Table3 : Lookup_n-D  NumberOfTableDimensions=1  BreakpointsForDimension1=Aeroparams.dh  Table=Aeroparams.ndh  InternalRulePriority=Speed  RndMeth=Simplest
  1-D Lookup Table4 : Lookup_n-D  NumberOfTableDimensions=1  BreakpointsForDimension1=Aeroparams.alpha  Table=Aeroparams.DCm  InternalRulePriority=Speed  RndMeth=Simplest
  2-D Lookup Table : Lookup_n-D  BreakpointsForDimension1=Aeroparams.alpha(1:14)  BreakpointsForDimension2=Aeroparams.beta  Table=Aeroparams.Cmlef  InternalRulePriority=Speed  RndMeth=Simplest
      settings: InputPortMap=u0,u1
  2-D Lookup Table1 : Lookup_n-D  BreakpointsForDimension1=Aeroparams.alpha  BreakpointsForDimension2=[Aeroparams.dh(1:4);15;20;25]  Table=Aeroparams.DCmds  InternalRulePriority=Speed  RndMeth=Simplest
      settings: InputPortMap=u0,u1
  3-D Lookup Table : Lookup_n-D  NumberOfTableDimensions=3  BreakpointsForDimension1=Aeroparams.alpha  BreakpointsForDimension2=Aeroparams.beta  BreakpointsForDimension3=Aeroparams.dh  Table=Aeroparams.Cm  InternalRulePriority=Speed  RndMeth=Simplest
      settings: InputPortMap=u0,u1,u2
  3-D Lookup Table1 : Lookup_n-D  NumberOfTableDimensions=3  BreakpointsForDimension1=Aeroparams.alpha  BreakpointsForDimension2=Aeroparams.beta  BreakpointsForDimension3=Aeroparams.dh  Table=Aeroparams.Cm  InternalRulePriority=Speed  RndMeth=Simplest
      settings: InputPortMap=u0,u1,u2
  Add : Sum  Inputs=-+
  Add1 : Sum  Inputs=+-
  Add2 : Sum  Inputs=+-
  Add3 : Sum
  Add4 : Sum  Inputs=+++++++
  Add5 : Sum  Inputs=+-
  Bus Selector1 : BusSelector  OutputSignals=elevator,speedbrake
  Bus Selector2 : BusSelector  OutputSignals=Vt,alpha,beta
  Bus Selector3 : BusSelector  OutputSignals=q
  Constant1 : Constant
  Constant3 : Constant  Value=0
  Constant4 : Constant
  Divide{,1..4,6..7} (7 alike) : Product  Inputs=**
  Divide5 : Product  Inputs=*/
  Gain : Gain  Gain=1/25
  Gain1 : Gain  Gain=1/60
  Gain2 : Gain  Gain=1/25
  Gain3 : Gain  Gain=2
  Radians to Degrees : simulink_extras/Transformations/Radians to Degrees
  Radians to Degrees1 : simulink_extras/Transformations/Radians to Degrees
  avoidzerodivision : Subsystem
  Cmt : Outport
  wires:
  actuatoraerooutputs/1 -> Bus Selector1/1
  vtalphabeta/1 -> Bus Selector2/1
  wb/1 -> Bus Selector3/1
  2-D Lookup Table/1 -> Add/2  "Cmlef"
  [dh0] -> 3-D Lookup Table1/3
  3-D Lookup Table1/1 -> Add/1  "Cmdh0"
  Constant1/1 -> Add1/1
  Gain/1 -> Add1/2
  Add/1 -> Divide/1
  Add1/1 -> Divide/2
  Bus Selector1/1 -> [elevator]  "<elevator>"
  Bus Selector1/2 -> [speedbrake]  "<speedbrake>"
  Bus Selector2/1 -> [Vt]  "<Vt>"
  Bus Selector2/2 -> Radians to Degrees/1  "<alpha>"
  Bus Selector2/3 -> Radians to Degrees1/1  "<beta>"
  Bus Selector3/1 -> [q]  "<q>"
  dlef/1 -> [dlef]
  cbar/1 -> [cbar]
  [alpha] -> 3-D Lookup Table/1
  [beta] -> 3-D Lookup Table/2
  [elevator] -> 3-D Lookup Table/3
  Constant3/1 -> [dh0]
  [beta] -> 3-D Lookup Table1/2
  [alpha] -> 3-D Lookup Table1/1
  [alpha] -> 2-D Lookup Table/1
  [beta] -> 2-D Lookup Table/2
  [dlef] -> Gain/1
  [alpha] -> 1-D Lookup Table/1
  [speedbrake] -> Gain1/1
  1-D Lookup Table/1 -> Divide3/1  "DCmsb"
  Gain1/1 -> Divide3/2
  [alpha] -> 1-D Lookup Table1/1
  [alpha] -> 1-D Lookup Table2/1
  [dlef] -> Gain2/1
  Gain2/1 -> Add2/2
  Constant4/1 -> Add2/1
  1-D Lookup Table2/1 -> Divide1/1  "DCmqlef"
  Add2/1 -> Divide1/2
  1-D Lookup Table1/1 -> Add3/1  "Cmq"
  Divide1/1 -> Add3/2
  Add3/1 -> Divide2/1
  [cbar] -> Divide4/1
  [q] -> Divide4/2
  [Vt] -> Gain3/1
  Divide4/1 -> Divide5/1
  Gain3/1 -> avoidzerodivision/1(in)
  Divide5/1 -> Divide2/2
  Add4/1 -> Cmt/1
  Czt/1 -> [Czt]
  [elevator] -> 1-D Lookup Table3/1
  3-D Lookup Table/1 -> Divide6/1  "Cm"
  1-D Lookup Table3/1 -> Divide6/2  "ndh"
  xcg/1 -> [xcg]
  xcgref/1 -> [xcgref]
  [Czt] -> Divide7/1
  [xcgref] -> Add5/1
  [xcg] -> Add5/2
  Add5/1 -> Divide7/2
  [alpha] -> 1-D Lookup Table4/1
  1-D Lookup Table4/1 -> Add4/6  "DCm"
  [alpha] -> 2-D Lookup Table1/1
  [elevator] -> 2-D Lookup Table1/2
  2-D Lookup Table1/1 -> Add4/7  "DCmds"
  Divide6/1 -> Add4/1
  Divide7/1 -> Add4/2
  Divide/1 -> Add4/3
  Divide3/1 -> Add4/4
  Divide2/1 -> Add4/5
  avoidzerodivision/1(out) -> Divide5/2
  Radians to Degrees/1 -> [alpha]
  Radians to Degrees1/1 -> [beta]

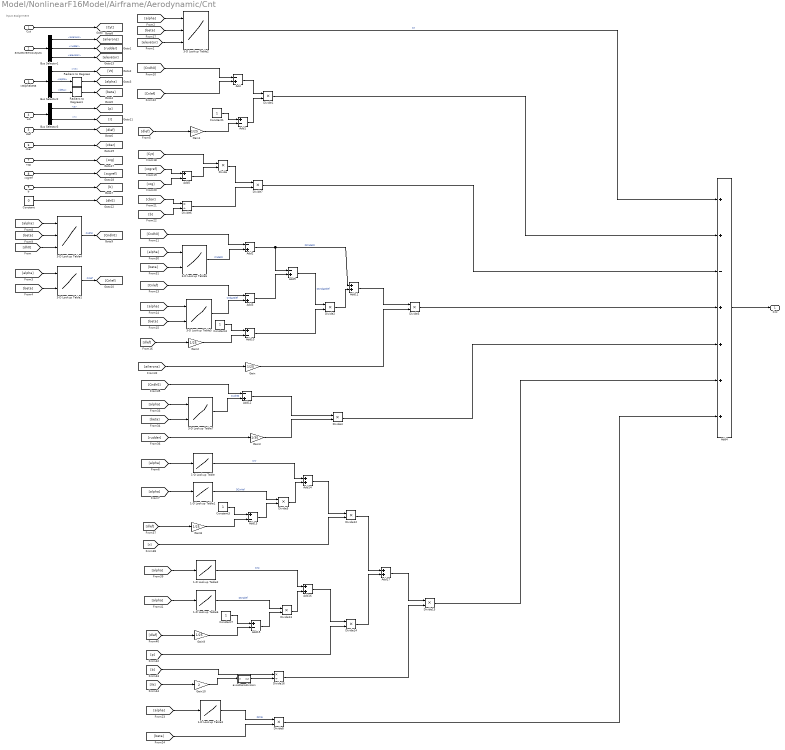
== system Model/NonlinearF16Model/Airframe/Aerodynamic/Cnt ==
  note: Input assignment
  Cyt : Inport
  actuatoraerooutputs : Inport  Port=2
  vtalphabeta : Inport  Port=3
  wb : Inport  Port=4
  dlef : Inport  Port=5
  cbar : Inport  Port=6
  xcg : Inport  Port=7
  xcgref : Inport  Port=8
  b : Inport  Port=9
  1-D Lookup Table : Lookup_n-D  NumberOfTableDimensions=1  BreakpointsForDimension1=Aeroparams.alpha  Table=Aeroparams.Cnr  InternalRulePriority=Speed  RndMeth=Simplest
  1-D Lookup Table1 : Lookup_n-D  NumberOfTableDimensions=1  BreakpointsForDimension1=Aeroparams.alpha(1:14)  Table=Aeroparams.DCnrlef  InternalRulePriority=Speed  RndMeth=Simplest
  1-D Lookup Table2 : Lookup_n-D  NumberOfTableDimensions=1  BreakpointsForDimension1=Aeroparams.alpha  Table=Aeroparams.Cnp  InternalRulePriority=Speed  RndMeth=Simplest
  1-D Lookup Table3 : Lookup_n-D  NumberOfTableDimensions=1  BreakpointsForDimension1=Aeroparams.alpha  Table=Aeroparams.DCnb  InternalRulePriority=Speed  RndMeth=Simplest
  1-D Lookup Table6 : Lookup_n-D  NumberOfTableDimensions=1  BreakpointsForDimension1=Aeroparams.alpha(1:14)  Table=Aeroparams.DCnplef  InternalRulePriority=Speed  RndMeth=Simplest
  3-D Lookup Table1 : Lookup_n-D  BreakpointsForDimension1=Aeroparams.alpha(1:14)  BreakpointsForDimension2=Aeroparams.beta  BreakpointsForDimension3=Aeroparams.dh  Table=Aeroparams.Cnlef  InternalRulePriority=Speed  RndMeth=Simplest
      settings: InputPortMap=u0,u1
  3-D Lookup Table2 : Lookup_n-D  NumberOfTableDimensions=3  BreakpointsForDimension1=Aeroparams.alpha  BreakpointsForDimension2=Aeroparams.beta  BreakpointsForDimension3=Aeroparams.dh([1 3 5])  Table=Aeroparams.Cn  InternalRulePriority=Speed  RndMeth=Simplest
      settings: InputPortMap=u0,u1,u2
  3-D Lookup Table4 : Lookup_n-D  NumberOfTableDimensions=3  BreakpointsForDimension1=Aeroparams.alpha  BreakpointsForDimension2=Aeroparams.beta  BreakpointsForDimension3=Aeroparams.dh([1 3 5])  Table=Aeroparams.Cn  InternalRulePriority=Speed  RndMeth=Simplest
      settings: InputPortMap=u0,u1,u2
  3-D Lookup Table5 : Lookup_n-D  BreakpointsForDimension1=Aeroparams.alpha(1:14)  BreakpointsForDimension2=Aeroparams.beta  BreakpointsForDimension3=Aeroparams.dh  Table=Aeroparams.Cnda20lef  InternalRulePriority=Speed  RndMeth=Simplest
      settings: InputPortMap=u0,u1
  3-D Lookup Table6 : Lookup_n-D  BreakpointsForDimension1=Aeroparams.alpha  BreakpointsForDimension2=Aeroparams.beta  BreakpointsForDimension3=Aeroparams.dh  Table=Aeroparams.Cnda20  InternalRulePriority=Speed  RndMeth=Simplest
      settings: InputPortMap=u0,u1
  3-D Lookup Table7 : Lookup_n-D  BreakpointsForDimension1=Aeroparams.alpha  BreakpointsForDimension2=Aeroparams.beta  BreakpointsForDimension3=Aeroparams.dh  Table=Aeroparams.Cndr30  InternalRulePriority=Speed  RndMeth=Simplest
      settings: InputPortMap=u0,u1
  Add{,2..3,9,12} (5 alike) : Sum  Inputs=-+
  Add{1,5,10,13,15} (5 alike) : Sum  Inputs=+-
  Add{11,14,16..17} (4 alike) : Sum
  Add4 : Sum  Inputs=++-++++
  Bus Selector1 : BusSelector  OutputSignals=ailerons,rudder,elevator
  Bus Selector2 : BusSelector  OutputSignals=Vt,alpha,beta
  Bus Selector3 : BusSelector  OutputSignals=p,r
  Constant : Constant  Value=0
  Constant{1,3..4,7} (4 alike) : Constant
  Divide{,1..5,7..8,12..15} (12 alike) : Product  Inputs=**
  Divide16 : Product  Inputs=*/
  Divide6 : Product  Inputs=*/
  Gain : Gain  Gain=1/20
  Gain{1..2,8..9} (4 alike) : Gain  Gain=1/25
  Gain10 : Gain  Gain=2
  Gain3 : Gain  Gain=1/30
  Radians to Degrees : simulink_extras/Transformations/Radians to Degrees
  Radians to Degrees1 : simulink_extras/Transformations/Radians to Degrees
  avoidzerodivision : Subsystem
  Cnt : Outport
  wires:
  Divide16/1 -> Divide15/2
  Gain10/1 -> avoidzerodivision/1(in)
  [Vt] -> Gain10/1
  [b] -> Divide16/1
  Add17/1 -> Divide15/1
  Divide14/1 -> Add17/2
  Divide12/1 -> Add17/1
  [p] -> Divide14/2
  Add16/1 -> Divide14/1
  [alpha] -> 1-D Lookup Table6/1
  Gain9/1 -> Add15/2
  Constant7/1 -> Add15/1
  [dlef] -> Gain9/1
  Add15/1 -> Divide13/2
  1-D Lookup Table6/1 -> Divide13/1  "DCnplef"
  Divide13/1 -> Add16/2
  [alpha] -> 1-D Lookup Table2/1
  1-D Lookup Table2/1 -> Add16/1  "Cnp"
  [r] -> Divide12/2
  Add14/1 -> Divide12/1
  Divide5/1 -> Add14/2
  1-D Lookup Table/1 -> Add14/1  "Cnr"
  1-D Lookup Table1/1 -> Divide5/1  "DCnrlef"
  Add13/1 -> Divide5/2
  [dlef] -> Gain8/1
  Constant3/1 -> Add13/1
  Gain8/1 -> Add13/2
  [alpha] -> 1-D Lookup Table1/1
  [alpha] -> 1-D Lookup Table/1
  Bus Selector3/2 -> [r]  "<r>"
  Gain3/1 -> Divide4/2
  Add12/1 -> Divide4/1
  [rudder] -> Gain3/1
  [Cndh0] -> Add12/1
  3-D Lookup Table7/1 -> Add12/2  "Cydr30"
  [alpha] -> 3-D Lookup Table7/1
  [beta] -> 3-D Lookup Table7/2
  Gain/1 -> Divide3/2
  [ailerons] -> Gain/1
  Add11/1 -> Divide3/1
  Divide2/1 -> Add11/2
  Gain2/1 -> Add10/2
  Constant4/1 -> Add10/1
  [dlef] -> Gain2/1
  Add10/1 -> Divide2/2
  Add9/1 -> Divide2/1  "DCnda20lef"
  [alpha] -> 3-D Lookup Table6/1
  [beta] -> 3-D Lookup Table6/2
  3-D Lookup Table6/1 -> Add2/2  "Cnda20"
  Add3/1 -> Add9/2
  Add2/1 -> Add11/1, Add9/1  "DCnda20"
  [beta] -> 3-D Lookup Table5/2
  [alpha] -> 3-D Lookup Table5/1
  3-D Lookup Table5/1 -> Add3/2  "Cnda20lef"
  [Cnlef] -> Add3/1
  3-D Lookup Table1/1 -> [Cnlef]  "Cnlef"
  [alpha] -> 3-D Lookup Table1/1
  [beta] -> 3-D Lookup Table1/2
  [Cndh0] -> Add2/1
  [Cndh0] -> Add/1
  3-D Lookup Table4/1 -> [Cndh0]  "Cndh0"
  [beta] -> 3-D Lookup Table4/2
  [alpha] -> 3-D Lookup Table4/1
  Add1/1 -> Divide1/2
  Add/1 -> Divide1/1
  [dlef] -> Gain1/1
  Constant1/1 -> Add1/1
  Gain1/1 -> Add1/2
  [Cnlef] -> Add/2
  actuatoraerooutputs/1 -> Bus Selector1/1
  vtalphabeta/1 -> Bus Selector2/1
  wb/1 -> Bus Selector3/1
  Bus Selector1/1 -> [ailerons]  "<ailerons>"
  Bus Selector1/2 -> [rudder]  "<rudder>"
  Bus Selector2/1 -> [Vt]  "<Vt>"
  Bus Selector2/2 -> Radians to Degrees/1  "<alpha>"
  Bus Selector2/3 -> Radians to Degrees1/1  "<beta>"
  Bus Selector3/1 -> [p]  "<p>"
  dlef/1 -> [dlef]
  b/1 -> [b]
  Add4/1 -> Cnt/1
  Cyt/1 -> [Cyt]
  Constant/1 -> [dh0]
  [dh0] -> 3-D Lookup Table4/3
  [elevator] -> 3-D Lookup Table2/3
  [alpha] -> 3-D Lookup Table2/1
  [beta] -> 3-D Lookup Table2/2
  Bus Selector1/3 -> [elevator]  "<elevator>"
  3-D Lookup Table2/1 -> Add4/1  "Cn"
  Divide1/1 -> Add4/2
  [xcgref] -> Add5/1
  [xcg] -> Add5/2
  [Cyt] -> Divide/1
  Add5/1 -> Divide/2
  [cbar] -> Divide6/1
  [b] -> Divide6/2
  Divide/1 -> Divide7/1
  Divide6/1 -> Divide7/2
  Divide7/1 -> Add4/3
  Divide3/1 -> Add4/4
  Divide4/1 -> Add4/5
  Divide15/1 -> Add4/6
  [alpha] -> 1-D Lookup Table3/1
  1-D Lookup Table3/1 -> Divide8/1  "DCnb"
  [beta] -> Divide8/2
  Divide8/1 -> Add4/7
  xcg/1 -> [xcg]
  cbar/1 -> [cbar]
  xcgref/1 -> [xcgref]
  avoidzerodivision/1(out) -> Divide16/2
  Radians to Degrees/1 -> [alpha]
  Radians to Degrees1/1 -> [beta]
